simulink model "simulator"  (Simulink 8.4)
settings: Solver=ode45  StartTime=0.0  StopTime=2880  RelTol=1e-3
values from neighbouring files (symbols this model uses):
  controllerFunction = @humanBolus    [simulator_setup.m]
  G0 = 0    [simulator_setup.m]
  GB = 4.5    [simulator_setup.m]
  I0 = 0.05    [simulator_setup.m]
  IB = IB0    (= 15)    [simulator_setup.m]
  MAX_AGE = 80    [simulator_setup.m]
  MEAL_B_CARBS = 50    [simulator_setup.m]
  MEAL_B_TIME = 480    [simulator_setup.m]
  MEAL_BYPASS = 0    [simulator_setup.m]
  MEAL_D_CARBS = 50    [simulator_setup.m]
  MEAL_D_TIME = 1050    [simulator_setup.m]
  MEAL_L_CARBS = 50    [simulator_setup.m]
  MEAL_L_TIME = 720    [simulator_setup.m]
  mealFunction = @mealNHanes    [simulator_setup.m]
  MEAN_BMI = 22    [simulator_setup.m]
  MIN_AGE = 5    [simulator_setup.m]
  N = .093    (= 0.093)    [simulator_setup.m]
  noiseFunction = @noiseBoth    [simulator_setup.m]
  P1 = .01    (= 0.01)    [simulator_setup.m]
  P2 = .025    (= 0.025)    [simulator_setup.m]
  P3 = 1.3*(10^-5)    (= 1.3e-05)    [simulator_setup.m]
  SWITCH_ARTIFICIAL_PANCREAS = 2    [simulator_setup.m]
  VI = 12    [simulator_setup.m]
  X0 = 0    [simulator_setup.m]
undefined symbols (not defined in the file or in its folder): flintmax, mealAbsorption
libraries: commrandsrc2 x2
settings Model: Creator=williammortl  LastModifiedBy=williammortl
settings DataIOCC: SignalLoggingSaveFormat=Dataset
settings OptimizationCC: ExpressionDepthLimit=128
settings DebuggingCC: UnderspecifiedInitializationDetection=Simplified  MergeDetectMultiDrivingBlocksExec=error  FcnCallInpInsideContextMsg=EnableAllAsError  StateNameClashWarn=none
settings GRTTargetCC: CombineOutputUpdateFcns=on  GRTInterface=off

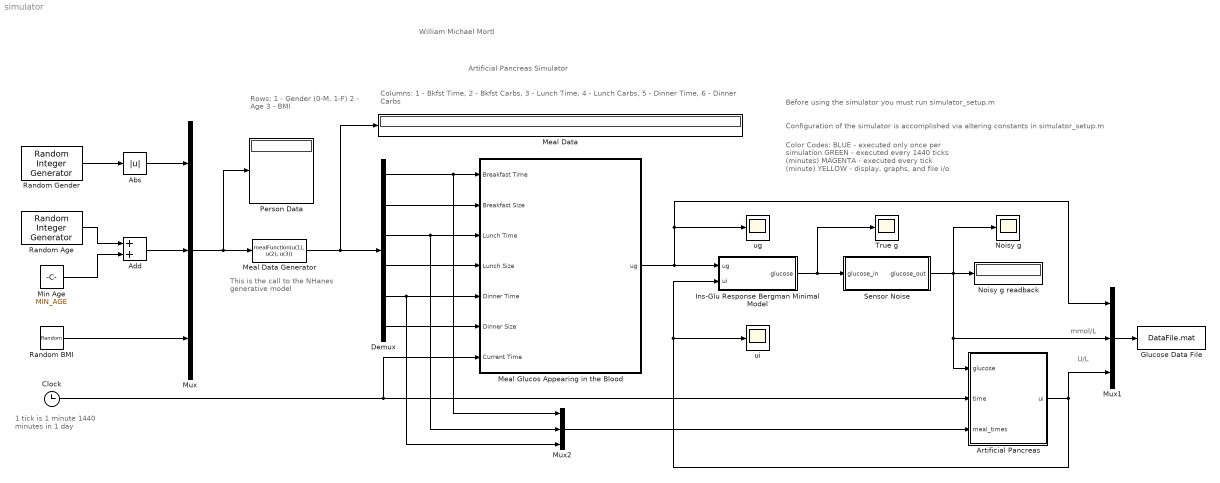
== system simulator ==
  note: Artificial Pancreas Simulator
  note: William Michael Mortl
  note: U/L
  note: mmol/L
  note: Before using the simulator you must run simulator_setup.m
  note: Color Codes:
      |
      | BLUE - executed only once per simulation
      | GREEN - executed every 1440 ticks (minutes)
      | MAGENTA - executed every tick (minute)
      | YELLOW - display, graphs, and file i/o
  note: Configuration of the simulator is accomplished via altering constants in simulator_setup.m
  note: Rows:
      |
      | 1 - Gender (0-M, 1-F)
      | 2 - Age
      | 3 - BMI
  note: This is the call to the NHanes
      | generative model
  note: Columns: 1 - Bkfst Time, 2 - Bkfst Carbs, 3 - Lunch Time, 4 - Lunch Carbs, 5 - Dinner Time, 6 - Dinner Carbs
  note: 1 tick is 1 minute
      | 1440 minutes in 1 day
  Abs : Abs
  Add : Sum
  Artificial Pancreas : Subsystem  SystemSampleTime=1
  Clock : Clock
  Demux : Demux  Outputs=6
  Glucose Data File : ToFile  Filename=DataFile.mat  SampleTime=1
  Ins-Glu Response Bergman Minimal Model : Subsystem  SystemSampleTime=1
  Meal Data : Display
  Meal Data Generator : MATLABFcn  MATLABFcn=mealFunction(u(1), u(2), u(3))  OutputDimensions=6  SampleTime=1440
  Meal Glucos Appearing in the Blood : Subsystem  TreatAsAtomicUnit=on  SystemSampleTime=1
  Min Age : Constant  Value=MIN_AGE
  Mux : Mux  Inputs=3
  Mux1 : Mux  Inputs=3
  Mux2 : Mux  Inputs=3
  Noisy g : Scope
      settings: YMin=-20  YMax=120  SaveName=ScopeData2
  Noisy g readback : Display
  Person Data : Display
  Random Age : commrandsrc2/Random Integer Generator  mul=MAX_AGE - MIN_AGE  seed=randi(777)  Ts=flintmax  frameBased=off  sampPerFrame=1  orient=off  outDataType=double
  Random BMI : RandomNumber  Mean=MEAN_BMI  Variance=5  SampleTime=flintmax
  Random Gender : commrandsrc2/Random Integer Generator  mul=2  seed=randi(777)  Ts=flintmax  frameBased=off  sampPerFrame=1  orient=off  outDataType=double
  Sensor Noise : Subsystem  SystemSampleTime=1
  True g : Scope
      settings: YMin=0  YMax=100
  ug : Scope
  ui : Scope
      settings: SaveName=ScopeData3
  wires:
  Meal Data Generator/1 -> Meal Data/1, Demux/1
  Mux/1 -> Person Data/1, Meal Data Generator/1
  Random Gender/1 -> Abs/1
  Add/1 -> Mux/2
  Random Age/1 -> Add/1
  Min Age/1 -> Add/2
  Random BMI/1 -> Mux/3
  Demux/1 -> Mux2/1, Meal Glucos Appearing in the Blood/1(Breakfast Time)
  Demux/2 -> Meal Glucos Appearing in the Blood/2(Breakfast Size)
  Demux/3 -> Mux2/2, Meal Glucos Appearing in the Blood/3(Lunch Time)
  Demux/4 -> Meal Glucos Appearing in the Blood/4(Lunch Size)
  Demux/5 -> Mux2/3, Meal Glucos Appearing in the Blood/5(Dinner Time)
  Demux/6 -> Meal Glucos Appearing in the Blood/6(Dinner Size)
  Meal Glucos Appearing in the Blood/1(ug) -> Ins-Glu Response Bergman Minimal Model/1(ug), Mux1/1, ug/1
  Artificial Pancreas/1(ui) -> Ins-Glu Response Bergman Minimal Model/2(ui), ui/1, Mux1/3
  Ins-Glu Response Bergman Minimal Model/1(glucose) -> True g/1, Sensor Noise/1(glucose_in)
  Clock/1 -> Meal Glucos Appearing in the Blood/7(Current Time), Artificial Pancreas/2(time)
  Abs/1 -> Mux/1
  Sensor Noise/1(glucose_out) -> Noisy g readback/1, Noisy g/1, Mux1/2, Artificial Pancreas/1(glucose)
  Mux1/1 -> Glucose Data File/1
  Mux2/1 -> Artificial Pancreas/3(meal_times)

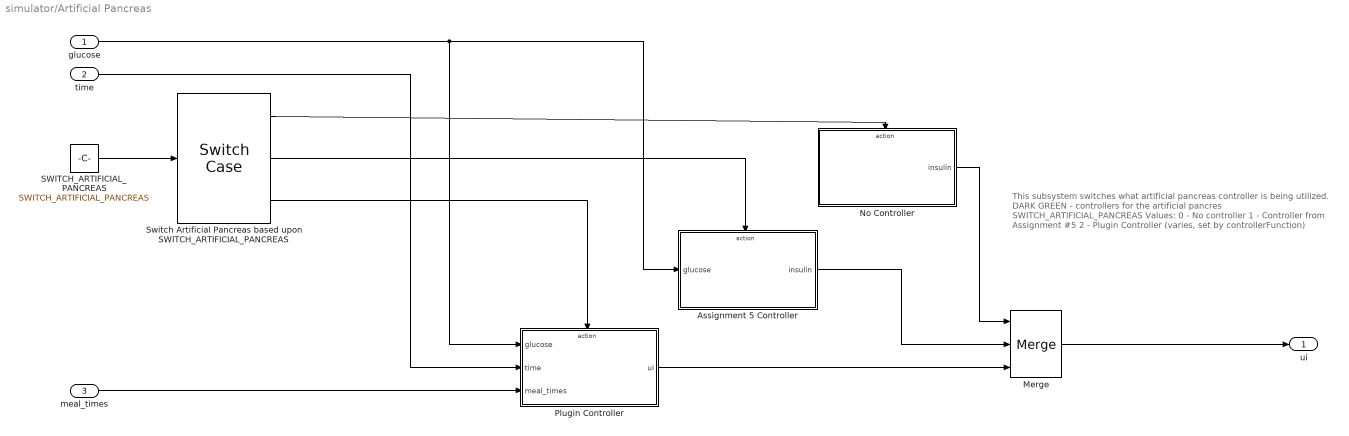
== system simulator/Artificial Pancreas ==
  note: This subsystem switches what artificial pancreas controller is being utilized.
      |
      | DARK GREEN - controllers for the artificial pancres
      |
      | SWITCH_ARTIFICIAL_PANCREAS Values:
      |
      | 0 - No controller
      | 1 - Controller from Assignment #5
      | 2 - Plugin Controller (varies, set by controllerFunction)
  glucose : Inport
  time : Inport  Port=2
  meal_times : Inport  Port=3
  Assignment 5 Controller : Subsystem  TreatAsAtomicUnit=on
  Merge : Merge  Inputs=3
  No Controller : Subsystem  TreatAsAtomicUnit=on
  Plugin Controller : Subsystem  TreatAsAtomicUnit=on
  SWITCH_ARTIFICIAL_PANCREAS : Constant  Value=SWITCH_ARTIFICIAL_PANCREAS
  "Switch Artificial Pancreas based upon SWITCH_ARTIFICIAL_PANCREAS " : SwitchCase  CaseConditions={0, 1, 2}  ShowDefaultCase=off  SampleTime=1
  ui : Outport
  wires:
  SWITCH_ARTIFICIAL_PANCREAS/1 -> "Switch Artificial Pancreas based upon SWITCH_ARTIFICIAL_PANCREAS "/1
  "Switch Artificial Pancreas based upon SWITCH_ARTIFICIAL_PANCREAS "/1 -> No Controller/Action
  "Switch Artificial Pancreas based upon SWITCH_ARTIFICIAL_PANCREAS "/2 -> Assignment 5 Controller/Action
  Assignment 5 Controller/1(insulin) -> Merge/2
  No Controller/1(insulin) -> Merge/1
  glucose/1 -> Assignment 5 Controller/1(glucose), Plugin Controller/1(glucose)
  Plugin Controller/1(ui) -> Merge/3
  "Switch Artificial Pancreas based upon SWITCH_ARTIFICIAL_PANCREAS "/3 -> Plugin Controller/Action
  time/1 -> Plugin Controller/2(time)
  Merge/1 -> ui/1
  meal_times/1 -> Plugin Controller/3(meal_times)

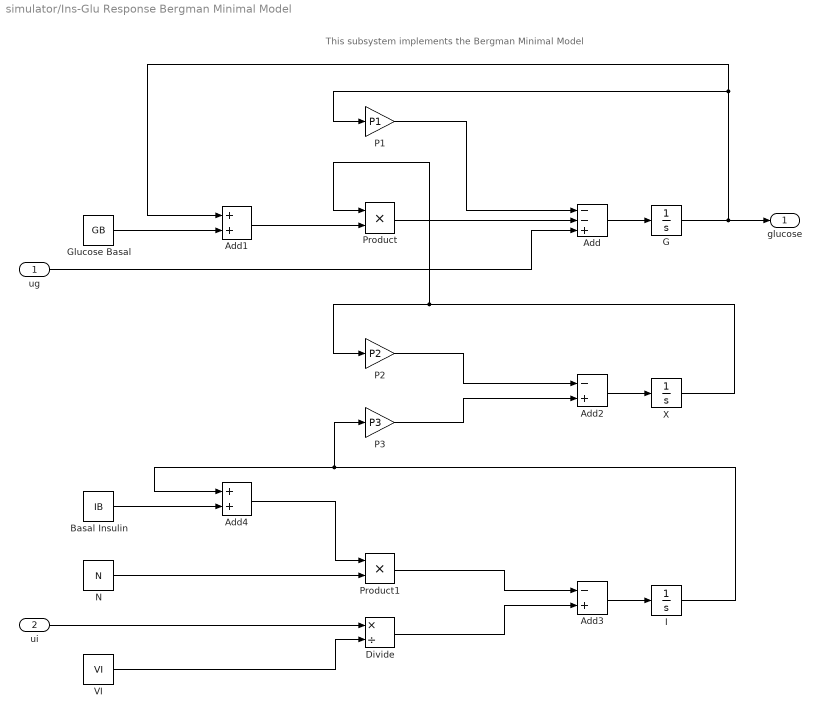
== system simulator/Ins-Glu Response Bergman Minimal Model ==
  note: This subsystem implements the Bergman Minimal Model
  ug : Inport
  ui : Inport  Port=2
  Add : Sum  Inputs=--+
  Add1 : Sum
  Add2 : Sum  Inputs=-+
  Add3 : Sum  Inputs=-+
  Add4 : Sum
  Basal Insulin : Constant  Value=IB
  Divide : Product  Inputs=*/
  G : Integrator  InitialCondition=G0
  Glucose Basal : Constant  Value=GB
  I : Integrator  InitialCondition=I0
  N : Constant  Value=N
  P1 : Gain  Gain=P1
  P2 : Gain  Gain=P2
  P3 : Gain  Gain=P3
  Product : Product
  Product1 : Product
  VI : Constant  Value=VI
  X : Integrator  InitialCondition=X0
  glucose : Outport
  wires:
  G/1 -> glucose/1, Add1/1, P1/1
  Add/1 -> G/1
  P1/1 -> Add/1
  X/1 -> Product/1, P2/1
  Product/1 -> Add/2
  Add1/1 -> Product/2
  Glucose Basal/1 -> Add1/2
  ug/1 -> Add/3
  Add2/1 -> X/1
  P2/1 -> Add2/1
  P3/1 -> Add2/2
  Add3/1 -> I/1
  N/1 -> Product1/2
  Product1/1 -> Add3/1
  Add4/1 -> Product1/1
  I/1 -> Add4/1, P3/1
  Basal Insulin/1 -> Add4/2
  Divide/1 -> Add3/2
  ui/1 -> Divide/1
  VI/1 -> Divide/2

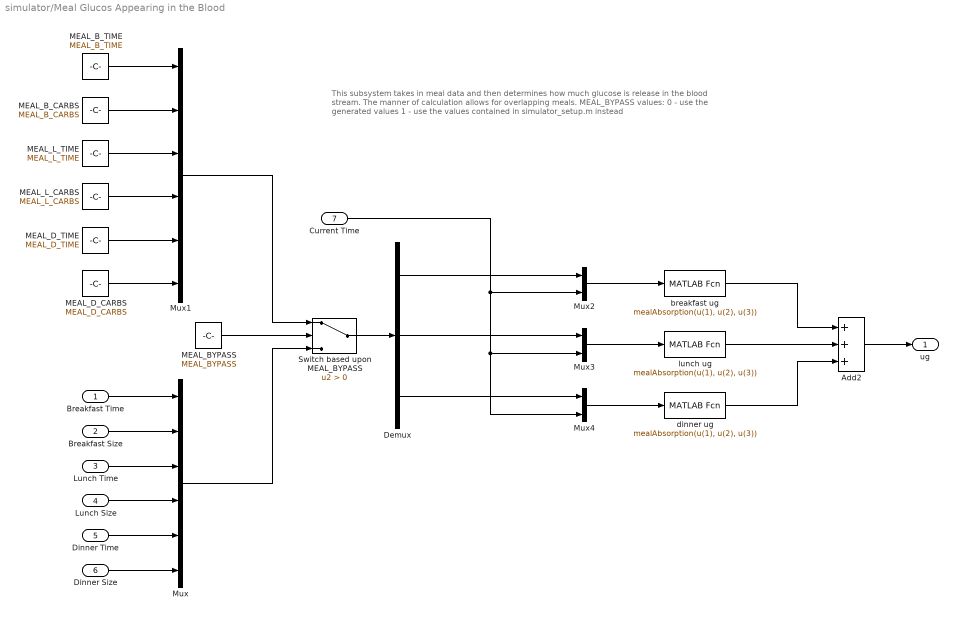
== system simulator/Meal Glucos Appearing in the Blood ==
  note: This subsystem takes in meal data and then determines how much glucose is release in the blood stream.
      | The manner of calculation allows for overlapping meals.
      |
      | MEAL_BYPASS values:
      | 0 - use the generated values
      | 1 - use the values contained in simulator_setup.m instead
  Breakfast Time : Inport
  Breakfast Size : Inport  Port=2
  Lunch Time : Inport  Port=3
  Lunch Size : Inport  Port=4
  Dinner Time : Inport  Port=5
  Dinner Size : Inport  Port=6
  Current Time : Inport  Port=7
  Add2 : Sum  Inputs=+++
  Demux : Demux  Outputs=3
  MEAL_BYPASS : Constant  Value=MEAL_BYPASS
  MEAL_B_CARBS : Constant  Value=MEAL_B_CARBS
  MEAL_B_TIME : Constant  Value=MEAL_B_TIME
  MEAL_D_CARBS : Constant  Value=MEAL_D_CARBS
  MEAL_D_TIME : Constant  Value=MEAL_D_TIME
  MEAL_L_CARBS : Constant  Value=MEAL_L_CARBS
  MEAL_L_TIME : Constant  Value=MEAL_L_TIME
  Mux : Mux  Inputs=6
  Mux1 : Mux  Inputs=6
  Mux2 : Mux  Inputs=2
  Mux3 : Mux  Inputs=2
  Mux4 : Mux  Inputs=2
  Switch based upon MEAL_BYPASS : Switch  Criteria=u2 > Threshold
  breakfast ug : MATLABFcn  MATLABFcn=mealAbsorption(u(1), u(2), u(3))  OutputDimensions=1
  dinner ug : MATLABFcn  MATLABFcn=mealAbsorption(u(1), u(2), u(3))  OutputDimensions=1
  lunch ug : MATLABFcn  MATLABFcn=mealAbsorption(u(1), u(2), u(3))  OutputDimensions=1
  ug : Outport
  wires:
  dinner ug/1 -> Add2/3
  lunch ug/1 -> Add2/2
  breakfast ug/1 -> Add2/1
  Add2/1 -> ug/1
  Breakfast Time/1 -> Mux/1
  Breakfast Size/1 -> Mux/2
  Lunch Time/1 -> Mux/3
  Lunch Size/1 -> Mux/4
  Dinner Time/1 -> Mux/5
  Dinner Size/1 -> Mux/6
  MEAL_B_TIME/1 -> Mux1/1
  MEAL_B_CARBS/1 -> Mux1/2
  MEAL_L_TIME/1 -> Mux1/3
  MEAL_L_CARBS/1 -> Mux1/4
  MEAL_D_TIME/1 -> Mux1/5
  MEAL_D_CARBS/1 -> Mux1/6
  MEAL_BYPASS/1 -> Switch based upon MEAL_BYPASS/2
  Mux1/1 -> Switch based upon MEAL_BYPASS/1
  Mux/1 -> Switch based upon MEAL_BYPASS/3
  Switch based upon MEAL_BYPASS/1 -> Demux/1
  Demux/1 -> Mux2/1
  Current Time/1 -> Mux4/2, Mux3/2, Mux2/2
  Demux/2 -> Mux3/1
  Demux/3 -> Mux4/1
  Mux2/1 -> breakfast ug/1
  Mux3/1 -> lunch ug/1
  Mux4/1 -> dinner ug/1

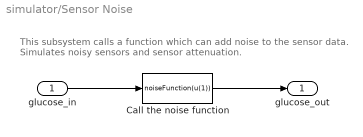
== system simulator/Sensor Noise ==
  note: This subsystem calls a function which can add noise to the sensor data.
      | Simulates noisy sensors and sensor attenuation.
  glucose_in : Inport
  Call the noise function : MATLABFcn  MATLABFcn=noiseFunction(u(1))  OutputDimensions=1
  glucose_out : Outport
  wires:
  glucose_in/1 -> Call the noise function/1
  Call the noise function/1 -> glucose_out/1

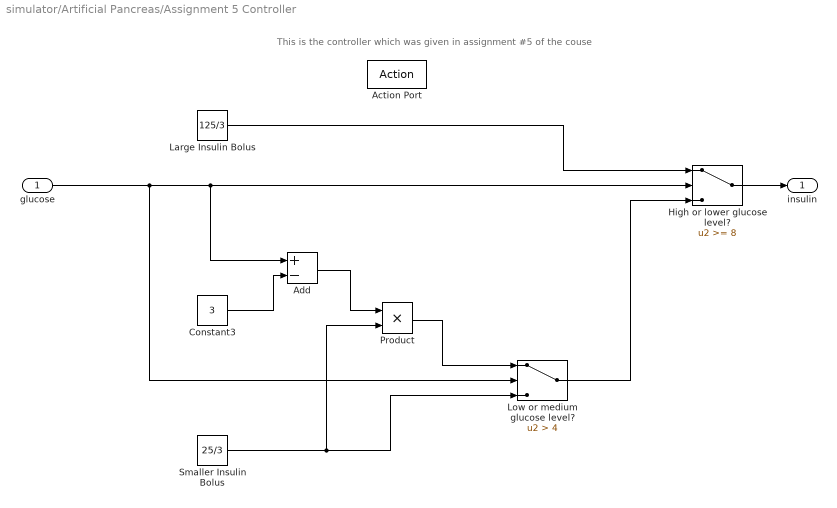
== system simulator/Artificial Pancreas/Assignment 5 Controller ==
  note: This is the controller which was given in assignment #5 of the couse
  glucose : Inport
  Action Port : ActionPort  ActionType=case
  Add : Sum  Inputs=+-
  Constant3 : Constant  Value=3
  High or lower glucose level? : Switch  Threshold=8
  Large Insulin Bolus : Constant  Value=125/3
  Low or medium glucose level? : Switch  Criteria=u2 > Threshold  Threshold=4
  Product : Product
  Smaller Insulin Bolus : Constant  Value=25/3
  insulin : Outport
  wires:
  Large Insulin Bolus/1 -> High or lower glucose level?/1
  glucose/1 -> Low or medium glucose level?/2, Add/1, High or lower glucose level?/2
  High or lower glucose level?/1 -> insulin/1
  Smaller Insulin Bolus/1 -> Low or medium glucose level?/3, Product/2
  Product/1 -> Low or medium glucose level?/1
  Low or medium glucose level?/1 -> High or lower glucose level?/3
  Constant3/1 -> Add/2
  Add/1 -> Product/1

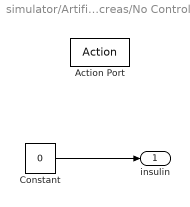
== system simulator/Artificial Pancreas/No Controller ==
  Action Port : ActionPort  ActionType=case
  Constant : Constant  Value=0
  insulin : Outport
  wires:
  Constant/1 -> insulin/1

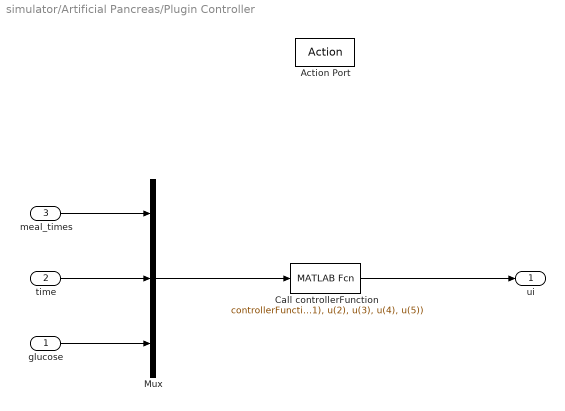
== system simulator/Artificial Pancreas/Plugin Controller ==
  glucose : Inport
  time : Inport  Port=2
  meal_times : Inport  Port=3
  Action Port : ActionPort  ActionType=case
  Call controllerFunction : MATLABFcn  MATLABFcn=controllerFunction(u(1), u(2), u(3), u(4), u(5))  OutputDimensions=1  Output1D=off  SampleTime=1
  Mux : Mux  Inputs=3
  ui : Outport
  wires:
  meal_times/1 -> Mux/1
  time/1 -> Mux/2
  glucose/1 -> Mux/3
  Mux/1 -> Call controllerFunction/1
  Call controllerFunction/1 -> ui/1
